simulink model "quasisq_wave"  (R2017a)
settings: Solver=VariableStepAuto  StartTime=0.0  StopTime=5  MaxStep=1e-4  RelTol=1e-3
libraries: powerlib x10, powerlib_meascontrol x2
settings Model: Creator=HP  LastModifiedBy=lenovo 520

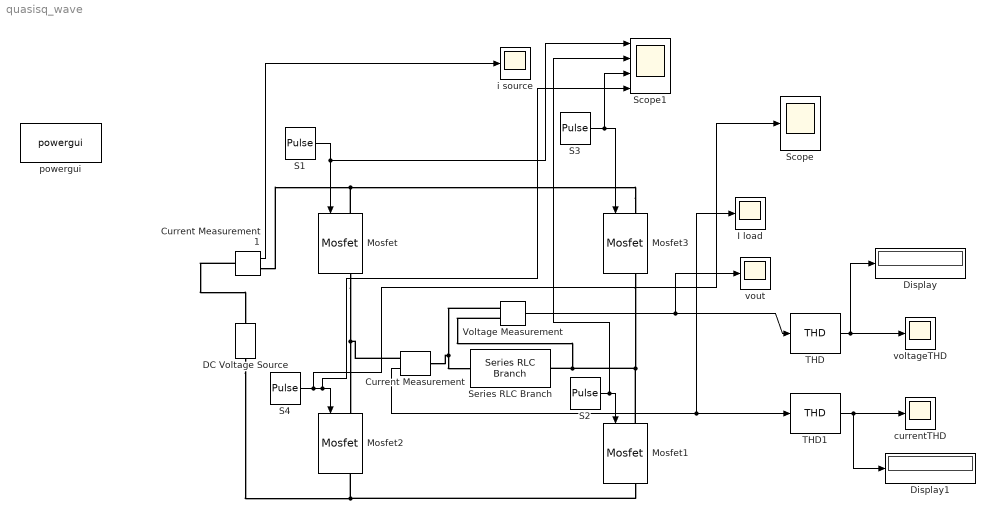
== system quasisq_wave ==
  Current Measurement : powerlib/Measurements/Current Measurement  PhasorSimulation=off  OutputType=Complex  PSBequivalent=0
  Current Measurement1 : powerlib/Measurements/Current Measurement  PhasorSimulation=off  OutputType=Complex  PSBequivalent=0
  DC Voltage Source : powerlib/Electrical Sources/DC Voltage Source  Amplitude=200  Measurements=None
  Display : Display
  Display1 : Display
  I load : Scope
  Mosfet{,1..3} (4 alike) : powerlib/Power Electronics/Mosfet  Ron=0.1  Lon=0  Rd=0.01  Vfd=0  IC=0  Rs=1e5  Cs=inf  Measurements=on
  S1 : DiscretePulseGenerator  PulseType=Time based  Period=20e-3  PulseWidth=50  PhaseDelay=2.5e-3
  S2 : DiscretePulseGenerator  PulseType=Time based  Period=20e-3  PulseWidth=50
  S3 : DiscretePulseGenerator  PulseType=Time based  Period=20e-3  PulseWidth=50  PhaseDelay=10e-3
  S4 : DiscretePulseGenerator  PulseType=Time based  Period=20e-3  PulseWidth=50  PhaseDelay=-7.5e-3
  Scope : Scope
  Scope1 : Scope  NumInputPorts=4
  Series RLC Branch : powerlib/Elements/Series RLC Branch  LConnTagsString=__new0  RConnTagsString=__new0  BranchType=RL  Resistance=1  Inductance=5e-3  SetiL0=off  InitialCurrent=0  Capacitance=1e-6  Setx0=off  InitialVoltage=0  Measurements=None
  THD : powerlib_meascontrol/Measurements/THD  Freq=50  Ts=0
  THD1 : powerlib_meascontrol/Measurements/THD  Freq=50  Ts=0
  Voltage Measurement : powerlib/Measurements/Voltage Measurement  PhasorSimulation=off  OutputType=Complex  PSBequivalent=0
  currentTHD : Scope
  i source : Scope
  powergui : powerlib/powergui  Priority=1  SimulationMode=Continuous  SampleTime=50e-6  frequency=60  Iterations=50  frequencyindice=0  Pbase=100e6  ErrMax=1e-4  UnitsV=kV  UnitsW=MW  buscounter=0  FunctionMessages=off  echomessages=off  EnableUseOfTLC=off  CurrentSourceSwitches=off  DisableSnubberDevices=off  DisableRonSwitches=off  DisableVfSwitches=off  DisplayEquations=off  SolverType=Tustin/Backward Euler (TBE)  Interpol=off  ExternalGateDelay=off  methode=off  Ts=100  x0status=blocks  SPID=on  SwTol=0  HookPort=off  RestoreLinks=warning  ResistiveCurrentMeasurement=off  Frange=[0:2:500]  Ylog=off  Xlog=on  ShowGrid=off  save=off  variable=ZData  structure=i3  ZoomFFT=off  StartTime=0.1  cycles=5  DisplayStyle=1  fundamental=50  FreqAxis=off  MaxFrequency=500  frequencyindicesteady=1  RmsSteady=1  display=off
  voltageTHD : Scope
  vout : Scope
  wires:
  THD1/1 -> Display1/1, currentTHD/1
  Current Measurement1/1 -> i source/1
  Current Measurement/1 -> I load/1, THD1/1
  S3/1 -> Scope1/3, Mosfet3/1
  THD/1 -> Display/1, voltageTHD/1
  S1/1 -> Scope1/1, Mosfet/1
  Voltage Measurement/1 -> vout/1, THD/1
  S4/1 -> Scope/1, Scope1/4, Mosfet2/1
  S2/1 -> Scope1/2, Mosfet1/1
  connections:
  Mosfet/RConn1 -- Current Measurement/RConn1 -- Mosfet2/LConn1
  Mosfet1/LConn1 -- Voltage Measurement/LConn2 -- Series RLC Branch/RConn1 -- Mosfet3/RConn1
  Voltage Measurement/LConn1 -- Current Measurement/LConn1 -- Series RLC Branch/LConn1
  Mosfet2/RConn1 -- Mosfet1/RConn1 -- DC Voltage Source/LConn1
  Mosfet3/LConn1 -- Mosfet/LConn1 -- Current Measurement1/RConn1
  Current Measurement1/LConn1 -- DC Voltage Source/RConn1
